simulink model "test1"  (R2021a)
settings: Solver=VariableStepAuto  StartTime=0.0  StopTime=10.0  MaxStep=te/50/10  RelTol=1e-3
values from neighbouring files (symbols this model uses):
  A = 9e-4    (= 0.0009)    [Electromagnet_par.m]    (also in coil_ironcore.m = 0.0005; sim21_ODE.m = 2)
  f = 50    [coil_ironcore.m]    (also in sim21_ODE.m = 1)
  phi = pi/4    (= 0.785398163397)    [sim21_ODE.m]
settings Model: Creator=ocean  LastModifiedBy=ocean

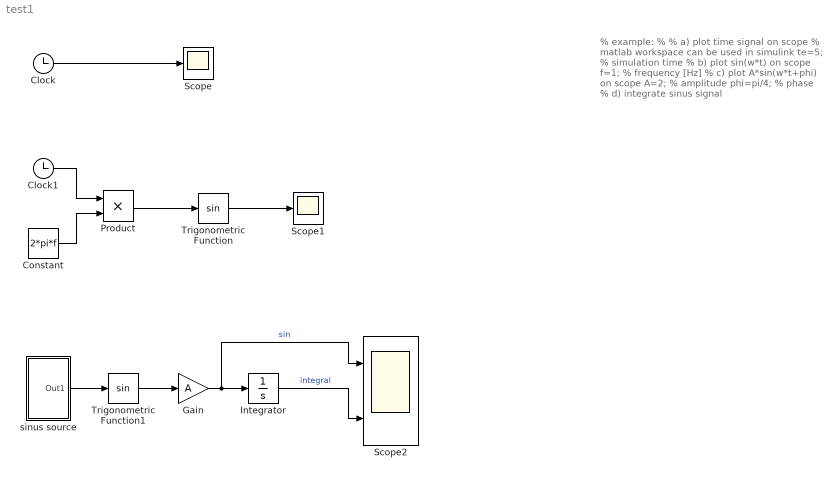
== system test1 ==
  note: % example:
      | %
      | % a) plot time signal on scope
      | % matlab workspace can be used in simulink
      | te=5;       % simulation time
      |
      | % b) plot sin(w*t) on scope
      | f=1;        % frequency [Hz]
      |
      | % c) plot A*sin(w*t+phi) on scope
      | A=2;        % amplitude
      | phi=pi/4;   % phase
      |
      | % d) integrate sinus signal
  Clock : Clock
  Clock1 : Clock
  Constant : Constant  Value=2*pi*f
  Gain : Gain  Gain=A
  Integrator : Integrator
  Product : Product
  Scope : Scope
  Scope1 : Scope
  Scope2 : Scope  NumInputPorts=2
  Trigonometric Function : Trigonometry
  Trigonometric Function1 : Trigonometry
  sinus source : Subsystem
  wires:
  Clock/1 -> Scope/1
  Clock1/1 -> Product/1
  Constant/1 -> Product/2
  Product/1 -> Trigonometric Function/1
  Trigonometric Function/1 -> Scope1/1
  Trigonometric Function1/1 -> Gain/1
  Gain/1 -> Scope2/1, Integrator/1  "sin"
  Integrator/1 -> Scope2/2  "integral"
  sinus source/1(Out1) -> Trigonometric Function1/1

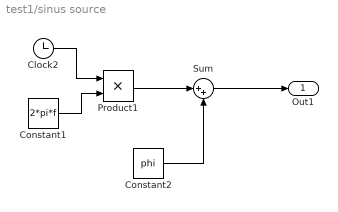
== system test1/sinus source ==
  Clock2 : Clock
  Constant1 : Constant  Value=2*pi*f
  Constant2 : Constant  Value=phi
  Product1 : Product
  Sum : Sum  Inputs=|++
  Out1 : Outport
  wires:
  Clock2/1 -> Product1/1
  Constant2/1 -> Sum/2
  Constant1/1 -> Product1/2
  Product1/1 -> Sum/1
  Sum/1 -> Out1/1
